simulink model "myfile"  (R2020a)
settings: Solver=ode4  StartTime=0.0  StopTime=inf  FixedStep=0.001  RelTol=1e-3
undefined symbols (not defined in the file or in its folder): National_Instruments, PCIe
libraries: sldrtlib x3
settings Model: Creator=me-clab2  LastModifiedBy=me-clab2
settings DataIOCC: SaveFormat=StructureWithTime
settings OptimizationCC: BlockReduction=off  OptimizeBlockIOStorage=off
settings RTWCC: Description=Simulink Desktop Real-Time  SystemTargetFile=sldrt.tlc  TemplateMakefile=sldrt.tmf  RTWCompilerOptimization=on
settings CodeAppCC: MaxIdLength=95
settings SimulinkDesktopRealTimeCC: TargetPreCompLibLocation=C:\Program Files\MATLAB\R2020a\toolbox\sldrt\lib\win64  TargetLangStandard=C89/C90 (ANSI)

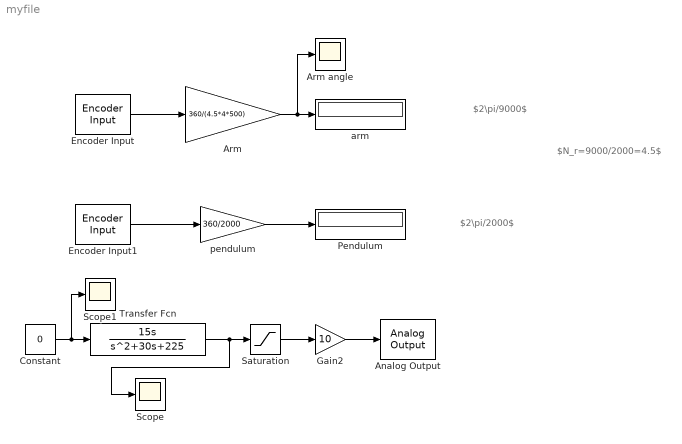
== system myfile ==
  note: $N_r=9000/2000=4.5$
  note: $2\pi/2000$
  note: $2\pi/9000$
  Analog Output : sldrtlib/Analog Output  SampleTime=0.001  MaxMissedTicks=10  ShowMissedTicks=off  YieldWhenWaiting=off  DrvName=National_Instruments/PCIe-6321  DrvAddress=4294967295  DrvOptions=[0 0 0 2 2 2 2]  Channels=[2]  RangeMode=1  VoltRange=1  InitialValue=0  FinalValue=0
      settings: AttributesFormatString=National Instruments\nPCIe-6321 [auto]
  Arm : Gain  Gain=360/(4.5*4*500)
  Arm angle : Scope
  Constant : Constant  Value=0
  Encoder Input : sldrtlib/Encoder Input  SampleTime=0.001  MaxMissedTicks=10  ShowMissedTicks=off  YieldWhenWaiting=off  DrvName=National_Instruments/PCIe-6321  DrvAddress=4294967295  DrvOptions=[0 0 0 2 2 2 2]  Channels=[1]  QuadMode=3  IndexPulse=1  InputFilter=Inf  DataType=1
      settings: AttributesFormatString=National Instruments\nPCIe-6321 [auto]
  Encoder Input1 : sldrtlib/Encoder Input  SampleTime=0.001  MaxMissedTicks=10  ShowMissedTicks=off  YieldWhenWaiting=off  DrvName=National_Instruments/PCIe-6321  DrvAddress=4294967295  DrvOptions=[0 0 0 2 2 2 2]  Channels=[2]  QuadMode=3  IndexPulse=1  InputFilter=Inf  DataType=1
      settings: AttributesFormatString=National Instruments\nPCIe-6321 [auto]
  Gain2 : Gain  Gain=10
  Pendulum : Display
  Saturation : Saturate  UpperLimit=1  LowerLimit=-1
  Scope : Scope
  Scope1 : Scope
  Transfer Fcn : TransferFcn  Numerator=[15 0]  Denominator=[1 30 225]
  arm : Display
  pendulum : Gain  Gain=360/2000
  wires:
  Transfer Fcn/1 -> Scope/1, Saturation/1
  Constant/1 -> Scope1/1, Transfer Fcn/1
  Saturation/1 -> Gain2/1
  pendulum/1 -> Pendulum/1
  Encoder Input/1 -> Arm/1
  Gain2/1 -> Analog Output/1
  Arm/1 -> Arm angle/1, arm/1
  Encoder Input1/1 -> pendulum/1
